simulink model "UAVUGV2"  (R2018a)
settings: Solver=VariableStepAuto  StartTime=0.0  StopTime=300  RelTol=1e-3
libraries: simulink x1
settings Model: Creator=wangluo  LastModifiedBy=wangluo

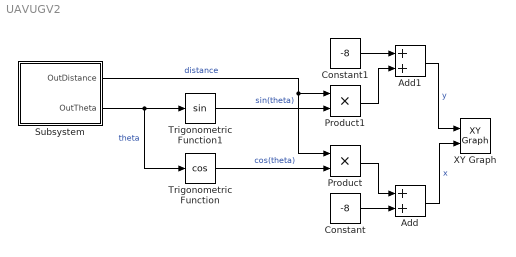
== system UAVUGV2 ==
  Add : Sum
  Add1 : Sum
  Constant : Constant  Value=-8
  Constant1 : Constant  Value=-8
  Product : Product
  Product1 : Product
  Subsystem : Subsystem
  Trigonometric Function : Trigonometry  Operator=cos
  Trigonometric Function1 : Trigonometry
  XY Graph : simulink/Sinks/XY Graph  xmin=-10  xmax=20  ymin=-10  ymax=15  st=-1
  wires:
  Subsystem/1(OutDistance) -> Product/1, Product1/1  "distance"
  Subsystem/2(OutTheta) -> Trigonometric Function1/1, Trigonometric Function/1  "theta"
  Trigonometric Function/1 -> Product/2  "cos(theta)"
  Trigonometric Function1/1 -> Product1/2  "sin(theta)"
  Product/1 -> Add/1
  Constant/1 -> Add/2
  Add/1 -> XY Graph/2  "x"
  Constant1/1 -> Add1/1
  Product1/1 -> Add1/2
  Add1/1 -> XY Graph/1  "y"

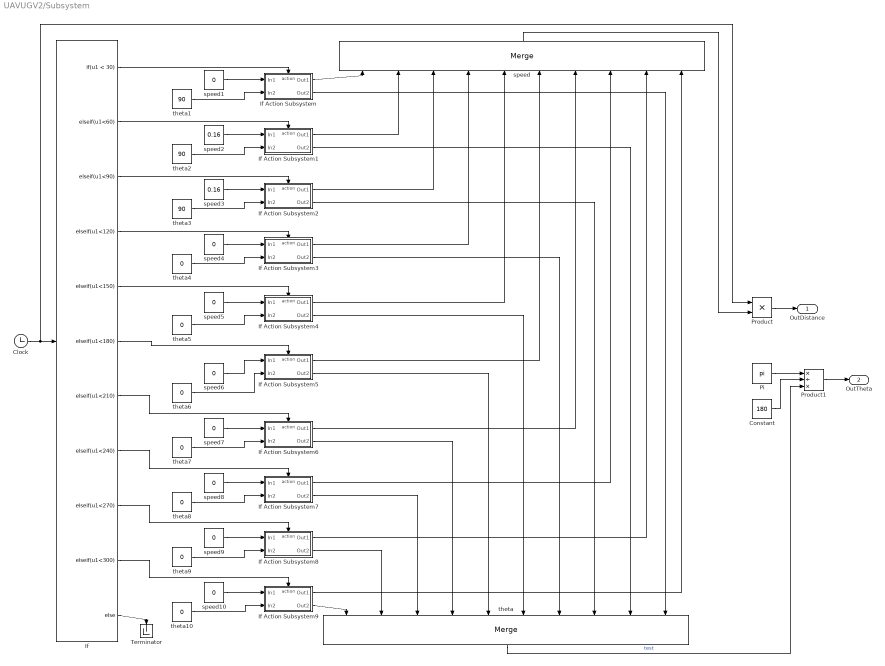
== system UAVUGV2/Subsystem ==
  Clock : Clock
      settings: Decimation=300
  Constant : Constant  Value=180
  If : If  IfExpression=u1 < 30  ElseIfExpressions=u1<60, u1<90, u1<120, u1<150, u1<180, u1<210, u1<240, u1<270, u1<300
  If Action Subsystem : Subsystem  TreatAsAtomicUnit=on
  If Action Subsystem1 : Subsystem  TreatAsAtomicUnit=on
  If Action Subsystem2 : Subsystem  TreatAsAtomicUnit=on
  If Action Subsystem3 : Subsystem  TreatAsAtomicUnit=on
  If Action Subsystem4 : Subsystem  TreatAsAtomicUnit=on
  If Action Subsystem5 : Subsystem  TreatAsAtomicUnit=on
  If Action Subsystem6 : Subsystem  TreatAsAtomicUnit=on
  If Action Subsystem7 : Subsystem  TreatAsAtomicUnit=on
  If Action Subsystem8 : Subsystem  TreatAsAtomicUnit=on
  If Action Subsystem9 : Subsystem  TreatAsAtomicUnit=on
  Pi : Constant  Value=pi
  Product : Product
  Product1 : Product  Inputs=*/*
  Terminator : Terminator
  speed : Merge  Inputs=10
  speed{1,4..10} (8 alike) : Constant  Value=0
  speed2 : Constant  Value=0.16
  speed3 : Constant  Value=0.16
  theta : Merge  Inputs=10
  theta1 : Constant  Value=90
  theta{4..10} (7 alike) : Constant  Value=0
  theta2 : Constant  Value=90
  theta3 : Constant  Value=90
  OutDistance : Outport
  OutTheta : Outport  Port=2
  wires:
  If Action Subsystem8/2(Out2) -> theta/2
  If Action Subsystem6/2(Out2) -> theta/4
  If Action Subsystem5/2(Out2) -> theta/5
  speed9/1 -> If Action Subsystem8/1(In1)
  speed8/1 -> If Action Subsystem7/1(In1)
  If Action Subsystem1/1(Out1) -> speed/2
  If Action Subsystem4/1(Out1) -> speed/5
  theta3/1 -> If Action Subsystem2/2(In2)
  If/10 -> If Action Subsystem9/Action
  If/4 -> If Action Subsystem3/Action
  If Action Subsystem2/2(Out2) -> theta/8
  speed4/1 -> If Action Subsystem3/1(In1)
  If/11 -> Terminator/1
  If Action Subsystem3/1(Out1) -> speed/4
  If Action Subsystem6/1(Out1) -> speed/7
  If Action Subsystem8/1(Out1) -> speed/9
  speed10/1 -> If Action Subsystem9/1(In1)
  If/2 -> If Action Subsystem1/Action
  If Action Subsystem2/1(Out1) -> speed/3
  If Action Subsystem9/1(Out1) -> speed/10
  speed1/1 -> If Action Subsystem/1(In1)
  theta6/1 -> If Action Subsystem5/2(In2)
  If/1 -> If Action Subsystem/Action
  If Action Subsystem/1(Out1) -> speed/1
  If Action Subsystem9/2(Out2) -> theta/1
  If Action Subsystem3/2(Out2) -> theta/7
  If Action Subsystem1/2(Out2) -> theta/9
  If Action Subsystem/2(Out2) -> theta/10
  theta7/1 -> If Action Subsystem6/2(In2)
  theta10/1 -> If Action Subsystem9/2(In2)
  If/9 -> If Action Subsystem8/Action
  If/7 -> If Action Subsystem6/Action
  Clock/1 -> If/1, Product/1
  speed3/1 -> If Action Subsystem2/1(In1)
  If/3 -> If Action Subsystem2/Action
  If Action Subsystem7/1(Out1) -> speed/8
  theta4/1 -> If Action Subsystem3/2(In2)
  theta9/1 -> If Action Subsystem8/2(In2)
  If/6 -> If Action Subsystem5/Action
  speed2/1 -> If Action Subsystem1/1(In1)
  speed6/1 -> If Action Subsystem5/1(In1)
  speed7/1 -> If Action Subsystem6/1(In1)
  theta2/1 -> If Action Subsystem1/2(In2)
  If Action Subsystem5/1(Out1) -> speed/6
  If/5 -> If Action Subsystem4/Action
  If Action Subsystem4/2(Out2) -> theta/6
  theta1/1 -> If Action Subsystem/2(In2)
  If/8 -> If Action Subsystem7/Action
  If Action Subsystem7/2(Out2) -> theta/3
  speed5/1 -> If Action Subsystem4/1(In1)
  theta8/1 -> If Action Subsystem7/2(In2)
  theta5/1 -> If Action Subsystem4/2(In2)
  speed/1 -> Product/2
  Pi/1 -> Product1/1
  Constant/1 -> Product1/2
  Product/1 -> OutDistance/1
  Product1/1 -> OutTheta/1
  theta/1 -> Product1/3  "test"

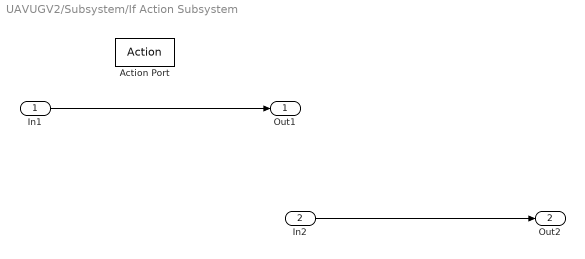
== system UAVUGV2/Subsystem/If Action Subsystem ==
  In1 : Inport
  In2 : Inport  Port=2
  Action Port : ActionPort  ActionType=then
  Out1 : Outport
  Out2 : Outport  Port=2
  wires:
  In1/1 -> Out1/1
  In2/1 -> Out2/1

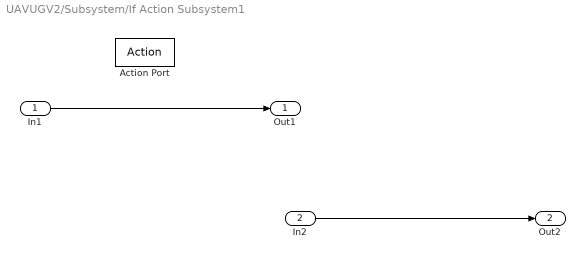
== system UAVUGV2/Subsystem/If Action Subsystem1 ==
  In1 : Inport
  In2 : Inport  Port=2
  Action Port : ActionPort  ActionType=elseif
  Out1 : Outport
  Out2 : Outport  Port=2
  wires:
  In1/1 -> Out1/1
  In2/1 -> Out2/1

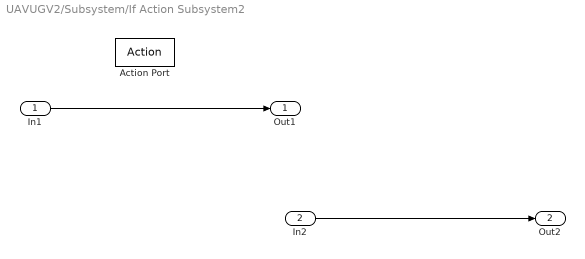
== system UAVUGV2/Subsystem/If Action Subsystem2 ==
  In1 : Inport
  In2 : Inport  Port=2
  Action Port : ActionPort  ActionType=elseif
  Out1 : Outport
  Out2 : Outport  Port=2
  wires:
  In1/1 -> Out1/1
  In2/1 -> Out2/1

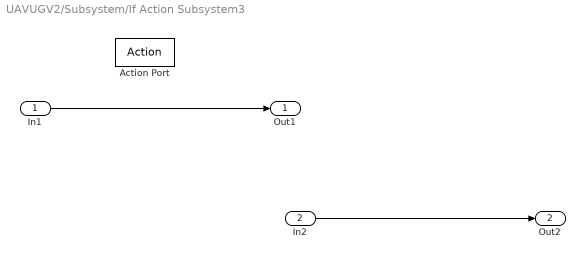
== system UAVUGV2/Subsystem/If Action Subsystem3 ==
  In1 : Inport
  In2 : Inport  Port=2
  Action Port : ActionPort  ActionType=elseif
  Out1 : Outport
  Out2 : Outport  Port=2
  wires:
  In1/1 -> Out1/1
  In2/1 -> Out2/1

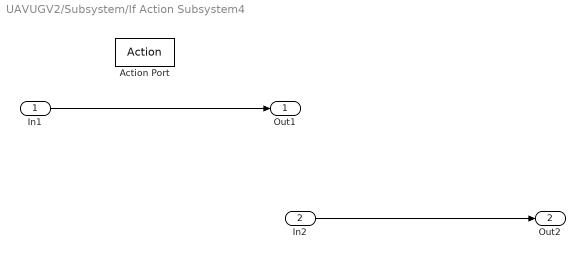
== system UAVUGV2/Subsystem/If Action Subsystem4 ==
  In1 : Inport
  In2 : Inport  Port=2
  Action Port : ActionPort  ActionType=elseif
  Out1 : Outport
  Out2 : Outport  Port=2
  wires:
  In1/1 -> Out1/1
  In2/1 -> Out2/1

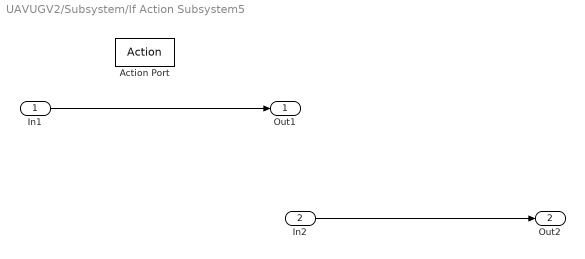
== system UAVUGV2/Subsystem/If Action Subsystem5 ==
  In1 : Inport
  In2 : Inport  Port=2
  Action Port : ActionPort  ActionType=elseif
  Out1 : Outport
  Out2 : Outport  Port=2
  wires:
  In1/1 -> Out1/1
  In2/1 -> Out2/1

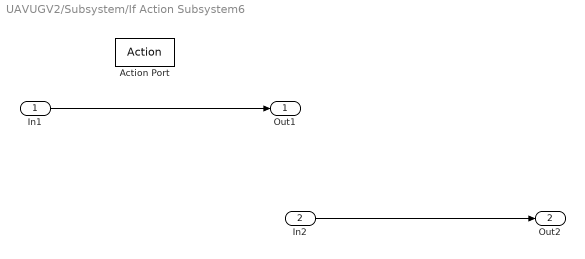
== system UAVUGV2/Subsystem/If Action Subsystem6 ==
  In1 : Inport
  In2 : Inport  Port=2
  Action Port : ActionPort  ActionType=elseif
  Out1 : Outport
  Out2 : Outport  Port=2
  wires:
  In1/1 -> Out1/1
  In2/1 -> Out2/1

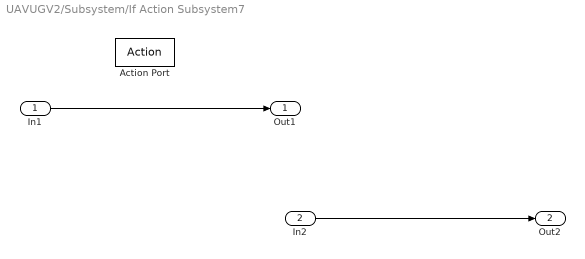
== system UAVUGV2/Subsystem/If Action Subsystem7 ==
  In1 : Inport
  In2 : Inport  Port=2
  Action Port : ActionPort  ActionType=elseif
  Out1 : Outport
  Out2 : Outport  Port=2
  wires:
  In1/1 -> Out1/1
  In2/1 -> Out2/1

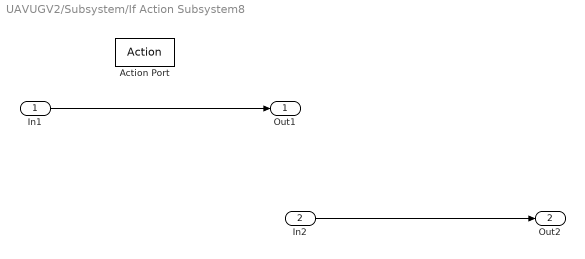
== system UAVUGV2/Subsystem/If Action Subsystem8 ==
  In1 : Inport
  In2 : Inport  Port=2
  Action Port : ActionPort  ActionType=elseif
  Out1 : Outport
  Out2 : Outport  Port=2
  wires:
  In1/1 -> Out1/1
  In2/1 -> Out2/1

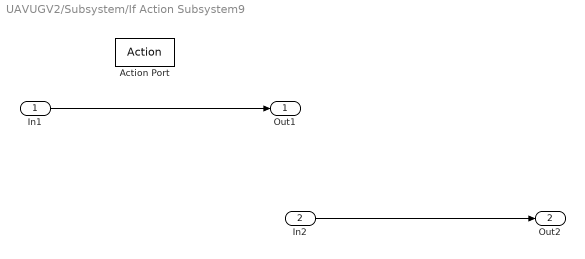
== system UAVUGV2/Subsystem/If Action Subsystem9 ==
  In1 : Inport
  In2 : Inport  Port=2
  Action Port : ActionPort  ActionType=elseif
  Out1 : Outport
  Out2 : Outport  Port=2
  wires:
  In1/1 -> Out1/1
  In2/1 -> Out2/1
